simulink library "thc"  (R2021b)
settings: Solver=VariableStepAuto  StartTime=0.0  StopTime=10.0  RelTol=1e-3
undefined symbols (not defined in the file or in its folder): ATHC_APTCQA_X_C, ATHC_APTCQB_X_C, ATHC_dAy_X_C, ATHC_Qeq_X_kmh, ATHC_VbaseC_X_C, ATHC_VbaseC_Y_W, ATHC_VbaseD_X_C, ATHC_VbaseH_X_C, FALSE, KTHC_ACMaxMinT_sec, KTHC_aDeice_K, KTHC_AGSDefLv_K, KTHC_AGSLv1_K, KTHC_AGSLv2_K, KTHC_AGSLv3_K, KTHC_AGSLv4_K, KTHC_AGSLv5_K, KTHC_AirIntUpdateT_sec, KTHC_APTCOneZoneMax_W, KTHC_APTCQMaxC_W, KTHC_APTCQminC_W, KTHC_APTCQminD_W, KTHC_APTCQminRe1_W, KTHC_APTCQminRe_W, KTHC_APTCQoffT_cnt, KTHC_APTCQonT_cnt, KTHC_APTCRiLeMaxDff_W, KTHC_APTCRiLeMinDff_W, KTHC_BatInTempDef_C, KTHC_bDeice_K, KTHC_CompMaxDeice_rpm, KTHC_CompMinDeice_rpm, KTHC_CompSotxvOp_K, KTHC_CompSotxvOpLow_rpm, KTHC_CompSpdmax_rpm, KTHC_CompSpdmaxBC1_rpm, KTHC_CompSpdmaxBC_rpm, KTHC_CompSpdmid1_rpm, KTHC_CompSpdmid2_rpm, KTHC_CompSpdmid3_rpm, KTHC_CompSpdmid_rpm, KTHC_CompSpdmin_rpm, KTHC_DAPTCQ1_W, KTHC_DAPTCQ2_W, KTHC_DAPTCQ3_W, KTHC_DcChSetTemp_C, KTHC_DehumidityEN_flg, KTHC_DeiceCycTime_K, KTHC_DTambSat1_C, KTHC_DTambSat2_C, KTHC_DTambsat3_C, KTHC_DTambsat4_C, KTHC_DTambSat5_C, KTHC_DTambSat_C, KTHC_DTcabin10_C, KTHC_DTCabin11_C, KTHC_DTcabin12_C, KTHC_DTcabin1_C, KTHC_DTcabin2_C, KTHC_DTcabin3_C ... (+347)
libraries: simulink x80
(part 4 of 8)

== system thc/THC/ThermalControl/AC/ModMath2 ==
  Dividend : Inport
  Divisor : Inport  Port=2
  Abs : Abs
  Constant : Constant  Value=eps
  Data Type Conversion : DataTypeConversion
  Data Type Conversion1 : DataTypeConversion
  Data Type Conversion2 : DataTypeConversion  OutDataTypeStr=single
  Divide : Product  Inputs=*/
  Equal : RelationalOperator  Operator=<=  OutDataTypeStr=boolean  RndMeth=Simplest
  Floor : Rounding
  Minus : Sum  Inputs=+-
  Product : Product
  Switch : Switch  Criteria=u2 > Threshold
  Remainder : Outport
  wires:
  Divisor/1 -> [Divisor]
  Equal/1 -> Switch/2
  Constant/1 -> Equal/2
  [Dividend] -> Divide/1
  Switch/1 -> Remainder/1
  [Dividend] -> Switch/1
  Minus/1 -> Switch/3
  Data Type Conversion2/1 -> Floor/1
  Data Type Conversion/1 -> Minus/2
  [Dividend] -> Minus/1
  Dividend/1 -> [Dividend]
  Floor/1 -> Data Type Conversion1/1
  Data Type Conversion1/1 -> Product/1
  [Divisor] -> Divide/2
  Abs/1 -> Equal/1
  [Divisor] -> Product/2
  Divide/1 -> Data Type Conversion2/1
  Product/1 -> Data Type Conversion/1
  [Divisor] -> Abs/1

== system thc/THC/ThermalControl/THCM_Conctrl/AGSandFan ==
  AGSLV : Inport
  Fan_Err : Inport  Port=2
  FAN : Inport  Port=3
  Compare To Constant : simulink/Logic and Bit Operations/Compare To Constant  relop=>  const=1  OutDataTypeStr=boolean
  Constant : Constant  Value=KTHC_AGSLv1_K
  Constant1 : Constant  Value=KTHC_AGSLv2_K
  Constant2 : Constant  Value=KTHC_AGSLv3_K
  Constant3 : Constant  Value=KTHC_AGSLv4_K
  Constant4 : Constant  Value=KTHC_AGSLv5_K
  Constant5 : Constant  Value=0
  Constant6 : Constant  Value=KTHC_AGSDefLv_K
  Constant7 : Constant  Value=KTHC_ErrHandleEN_flg
  Logical Operator : Logic  Inputs=3  AllPortsSameDT=off  OutDataTypeStr=boolean
  Multiport Switch : MultiPortSwitch  Inputs=6  DiagnosticForDefault=None
  Switch : Switch  Criteria=u2 > Threshold
  AGSOut : Outport
  wires:
  Constant2/1 -> Multiport Switch/4
  Constant1/1 -> Multiport Switch/3
  Constant/1 -> Multiport Switch/2
  Constant3/1 -> Multiport Switch/5
  Constant4/1 -> Multiport Switch/6
  Constant5/1 -> Multiport Switch/7
  AGSLV/1 -> Multiport Switch/1
  FAN/1 -> Compare To Constant/1
  Fan_Err/1 -> Logical Operator/1
  Compare To Constant/1 -> Logical Operator/2
  Multiport Switch/1 -> Switch/3
  Logical Operator/1 -> Switch/2
  Switch/1 -> AGSOut/1
  Constant6/1 -> Switch/1
  Constant7/1 -> Logical Operator/3

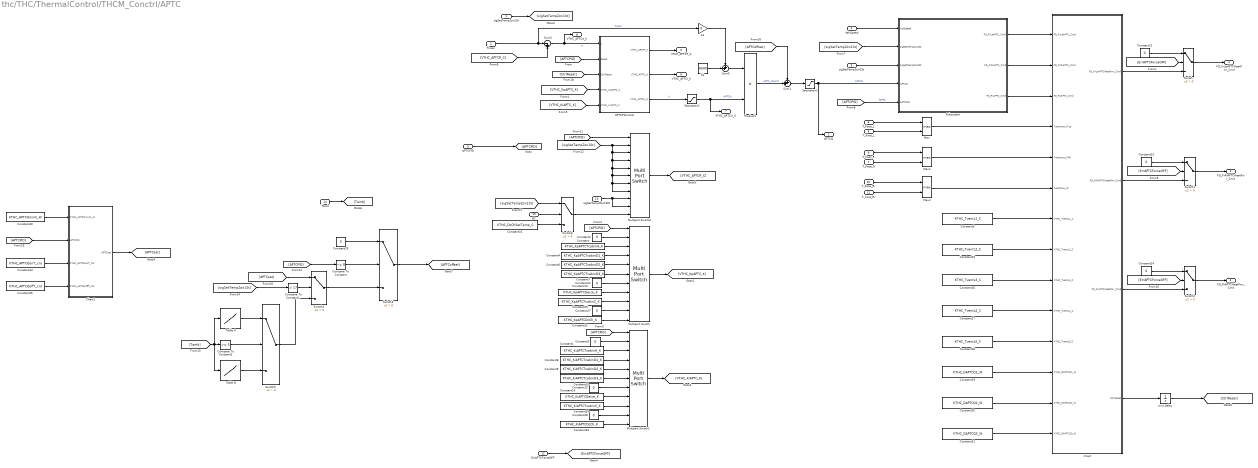
== system thc/THC/ThermalControl/THCM_Conctrl/APTC ==
  sigSetTempZon1St : Inport
  Tincar : Inport  Port=2
  APTCPID : Inport  Port=3
  VehSpeed : Inport  Port=4
  sigSetTempZon2St : Inport  Port=5
  T_Face_L : Inport  Port=6
  T_Face_R : Inport  Port=7
  T_Foot_L : Inport  Port=8
  T_Foot_R : Inport  Port=9
  T_Face_Rr : Inport  Port=10
  T_Foot_Rr : Inport  Port=11
  ErrAPTCForceOFF : Inport  Port=12
  sigSetTempZon1StC : Inport  Port=13
  Tamb : Inport  Port=14
  AC : Inport  Port=15
  APTCPIControl : Subsystem
  Chart : Stateflow chart  TreatAsAtomicUnit=on
  Chart1 : Stateflow chart  TreatAsAtomicUnit=on
  Compare To Constant : simulink/Logic and Bit Operations/Compare To Constant  relop=~=  const=8  OutDataTypeStr=boolean
  Compare To Constant1 : simulink/Logic and Bit Operations/Compare To Constant  relop=>  const=17  OutDataTypeStr=boolean
  Compare To Constant2 : simulink/Logic and Bit Operations/Compare To Constant  relop=>=  const=5  OutDataTypeStr=boolean
  Constant : Constant  Value=KTHC_KpAPTCTcabinH_K
  Constant1 : Constant  Value=KTHC_KiAPTCTcabinH_K
  Constant10 : Constant  Value=KTHC_KiAPTCTcabinD3_K
  Constant{2..3,11..12,22..24,27..29} (10 alike) : Constant  Value=0
  Constant13 : Constant  Value=KTHC_KpAPTCDeice_K
  Constant14 : Constant  Value=KTHC_KiAPTCDeice_K
  Constant15 : Constant  Value=KTHC_TventL2_C
  Constant16 : Constant  Value=KTHC_TventL3_C
  Constant17 : Constant  Value=KTHC_TventL4_C
  Constant18 : Constant  Value=KTHC_TventL5_C
  Constant19 : Constant  Value=KTHC_DAPTCQ1_W
  Constant20 : Constant  Value=KTHC_DAPTCQ2_W
  Constant21 : Constant  Value=KTHC_DAPTCQ3_W
  Constant25 : Constant  Value=KTHC_KpAPTCTcabinC_K
  Constant26 : Constant  Value=KTHC_KiAPTCTcabinC_K
  Constant30 : Constant  Value=KTHC_APTCQminC_W
  Constant31 : Constant  Value=KTHC_DcChSetTemp_C
  Constant32 : Constant  Value=KTHC_KpAPTCDcCh_K
  Constant33 : Constant  Value=KTHC_KiAPTCDcCh_K
  Constant34 : Constant  Value=KTHC_APTCQonT_cnt
  Constant35 : Constant  Value=KTHC_APTCQoffT_cnt
  Constant4 : Constant  Value=KTHC_KpAPTCTcabinD1_K
  Constant5 : Constant  Value=KTHC_TventL1_C
  Constant6 : Constant  Value=KTHC_KpAPTCTcabinD2_K
  Constant7 : Constant  Value=KTHC_KpAPTCTcabinD3_K
  Constant8 : Constant  Value=KTHC_KiAPTCTcabinD1_K
  Constant9 : Constant  Value=KTHC_KiAPTCTcabinD2_K
  Max : MinMax  Function=max  Inputs=2
  Max1 : MinMax  Function=max  Inputs=2
  Max2 : MinMax  Function=max  Inputs=2
  Multiport Switch : MultiPortSwitch  DataPortOrder=Zero-based contiguous  Inputs=10  zeroidx=on
  Multiport Switch1 : MultiPortSwitch  DataPortOrder=Zero-based contiguous  Inputs=10  zeroidx=on
  Multiport Switch2 : MultiPortSwitch  DataPortOrder=Zero-based contiguous  Inputs=10  zeroidx=on
  Product1 : Product
  Saturation1 : Saturate  UpperLimit=1  LowerLimit=0
  Saturation2 : Saturate  UpperLimit=6500  LowerLimit=0
  Subsystem : Subsystem
  Sum1 : Sum  Inputs=++|
  Sum3 : Sum  Inputs=|-+
  Sum5 : Sum  Inputs=++|
  Switch{,1..6} (7 alike) : Switch  Criteria=u2 > Threshold
  Table A : Lookup_n-D  NumberOfTableDimensions=1  BreakpointsForDimension1=ATHC_APTCQA_X_C  Table=MTHC_APTCQA_Y_W  InternalRulePriority=Speed  RndMeth=Simplest  InputSameDT=on
  Table B : Lookup_n-D  NumberOfTableDimensions=1  BreakpointsForDimension1=ATHC_APTCQB_X_C  Table=MTHC_APTCQB_Y_W  InternalRulePriority=Speed  RndMeth=Simplest  InputSameDT=on
  Unit Delay : UnitDelay  SampleTime=-1  HasFrameUpgradeWarning=on
  a1 : Gain  Gain=0
  b1 : Constant  Value=6500
  APTCQ : Outport
  FD_FrLeAPTCHeatPwr_Cmd : Outport  Port=2
  FD_FrRiAPTCHeatPwr_Cmd : Outport  Port=3
  FD_RrAPTCHeatPwr_Cmd : Outport  Port=4
  VTHC_APTCP_K : Outport  Port=5
  VTHC_APTCI_K : Outport  Port=6
  VTHC_APTCU_K : Outport  Port=7
  VTHC_APTCe_K : Outport  Port=8
  wires:
  [VTHC_APTCR_C] -> Sum3/2
  a1/1 -> Sum5/1
  Product1/1 -> Sum1/2  "APTC_nolimit"
  Saturation1/1 -> VTHC_APTCU_K/1, Product1/2  "APTC%"
  Tincar/1 -> a1/1, Sum3/1  "Tincar"
  Sum5/1 -> Product1/1
  b1/1 -> Sum5/2
  Sum3/1 -> VTHC_APTCe_K/1, APTCPIControl/1(x)  "e"
  APTCPIControl/3(VTHC_APTCU_K) -> Saturation1/1  "U"
  [APTCPID] -> APTCPIControl/2(Reset)
  Saturation2/1 -> APTCQ/1, Subsystem/4(APTCQ)  "APTCQ"
  Constant/1 -> Multiport Switch/3
  Constant1/1 -> Multiport Switch1/3
  APTCPIControl/1(VTHC_APTCP_K) -> VTHC_APTCP_K/1
  APTCPIControl/2(VTHC_APTCI_K) -> VTHC_APTCI_K/1
  [APTCPID] -> Multiport Switch/1
  Constant2/1 -> Multiport Switch/2
  Multiport Switch/1 -> [VTHC_KpAPTC_K]
  Multiport Switch1/1 -> [VTHC_KiAPTC_K]
  Constant3/1 -> Multiport Switch1/2
  [APTCPID] -> Multiport Switch1/1
  Constant4/1 -> Multiport Switch/4
  Constant6/1 -> Multiport Switch/5
  Constant7/1 -> Multiport Switch/6
  Constant8/1 -> Multiport Switch1/4
  Constant9/1 -> Multiport Switch1/5
  Constant10/1 -> Multiport Switch1/6
  [VTHC_KpAPTC_K] -> APTCPIControl/4(VTHC_KpAPTC_K)
  [VTHC_KiAPTC_K] -> APTCPIControl/5(VTHC_KiAPTC_K)
  Constant11/1 -> Multiport Switch/7
  Constant12/1 -> Multiport Switch1/7
  VehSpeed/1 -> Subsystem/1(VehSpeed)
  sigSetTempZon2St/1 -> Subsystem/3(sigSetTempZon2St)
  [sigSetTempZon1St] -> Subsystem/2(sigSetTempZon1St)
  sigSetTempZon1St/1 -> [sigSetTempZon1St]
  [APTCPID] -> Subsystem/5(APTCPID)  "fAPTC"
  Constant13/1 -> Multiport Switch/8
  Constant14/1 -> Multiport Switch1/8
  T_Face_Rr/1 -> Max2/1
  T_Foot_L/1 -> Max/2
  T_Face_L/1 -> Max/1
  T_Foot_R/1 -> Max1/1
  T_Face_R/1 -> Max1/2
  T_Foot_Rr/1 -> Max2/2
  Max/1 -> Chart/4(Tventmax_FrLe)
  Subsystem/1(FD_FrLeAPTC_Cmd) -> Chart/1(FD_FrLeAPTC_Cmd)
  Subsystem/2(FD_FrRiAPTC_Cmd) -> Chart/2(FD_FrRiAPTC_Cmd)
  Subsystem/3(FD_RrAPTC_Cmd) -> Chart/3(FD_RrAPTC_Cmd)
  Max1/1 -> Chart/5(Tventmax_FrRi)
  Max2/1 -> Chart/6(Tventmax_Rr)
  Constant5/1 -> Chart/7(KTHC_TventL1_C)
  Constant15/1 -> Chart/8(KTHC_TventL2_C)
  Constant16/1 -> Chart/9(KTHC_TventL3_C)
  Constant17/1 -> Chart/10(KTHC_TventL4_C)
  Constant18/1 -> Chart/11(KTHC_TventL5_C)
  Constant19/1 -> Chart/12(KTHC_DAPTCQ1_W)
  Constant20/1 -> Chart/13(KTHC_DAPTCQ2_W)
  Constant21/1 -> Chart/14(KTHC_DAPTCQ3_W)
  Chart/1(FD_FrLeAPTCHeatPwr_Cmd) -> Switch/3
  ErrAPTCForceOFF/1 -> [ErrAPTCForceOFF]
  Switch/1 -> FD_FrLeAPTCHeatPwr_Cmd/1
  [ErrAPTCForceOFF] -> Switch/2
  Constant22/1 -> Switch/1
  Constant23/1 -> Switch1/1
  [ErrAPTCForceOFF] -> Switch1/2
  Chart/2(FD_FrRiAPTCHeatPwr_Cmd) -> Switch1/3
  Switch1/1 -> FD_FrRiAPTCHeatPwr_Cmd/1
  Chart/3(FD_RrAPTCHeatPwr_Cmd) -> Switch2/3
  [ErrAPTCForceOFF] -> Switch2/2
  Constant24/1 -> Switch2/1
  Switch2/1 -> FD_RrAPTCHeatPwr_Cmd/1
  Multiport Switch2/1 -> [VTHC_APTCR_C]
  [APTCPID] -> Multiport Switch2/1
  [sigSetTempZon1St] -> Multiport Switch2/8, Multiport Switch2/7, Multiport Switch2/6, Multiport Switch2/5, Multiport Switch2/4, Multiport Switch2/3, Multiport Switch2/2
  Constant25/1 -> Multiport Switch/9
  Constant26/1 -> Multiport Switch1/9
  APTCPID/1 -> [APTCPID]
  sigSetTempZon1StC/1 -> Multiport Switch2/10, Multiport Switch2/9
  Constant27/1 -> Multiport Switch/10
  Constant28/1 -> Multiport Switch1/10
  [APTCPID] -> Compare To Constant/1
  [sigSetTempZon1St] -> Compare To Constant1/1
  Compare To Constant1/1 -> Switch4/2
  Compare To Constant/1 -> Switch3/2
  Constant29/1 -> Switch3/1
  Switch4/1 -> Switch3/3
  Tamb/1 -> [Tamb]
  [Tamb] -> Table B/1, Table A/1, Compare To Constant2/1
  Compare To Constant2/1 -> Switch5/2
  Table A/1 -> Switch5/1
  Table B/1 -> Switch5/3
  Switch5/1 -> Switch4/3
  Switch3/1 -> [APTCoffset]
  Sum1/1 -> Saturation2/1
  [APTCoffset] -> Sum1/1
  AC/1 -> Switch6/2
  [sigSetTempZon1St] -> Switch6/1
  Constant31/1 -> Switch6/3
  Switch6/1 -> Multiport Switch2/11
  Constant32/1 -> Multiport Switch/11
  Constant33/1 -> Multiport Switch1/11
  Chart/4(CtrlReset) -> Unit Delay/1
  Unit Delay/1 -> [CtrlReset]
  [CtrlReset] -> APTCPIControl/3(CtrlReset)
  Constant30/1 -> Chart1/1(KTHC_APTCQminC_W)
  [APTCPID] -> Chart1/2(APTCPID)
  Constant34/1 -> Chart1/3(KTHC_APTCQonT_cnt)
  Constant35/1 -> Chart1/4(KTHC_APTCQoffT_cnt)
  Chart1/1(APTCset) -> [APTCset]
  [APTCset] -> Switch4/1

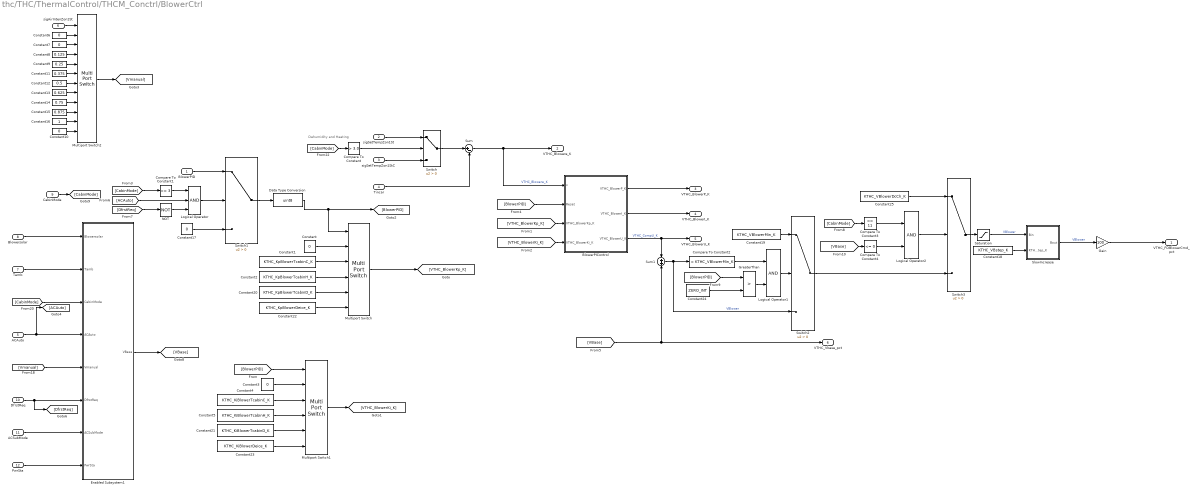
== system thc/THC/ThermalControl/THCM_Conctrl/BlowerCtrl ==
  note: Dehumidity and Heating
  BlowerPID : Inport
  sigSetTempZon1St : Inport  Port=2
  sigSetTempZon1StC : Inport  Port=3
  Tincar : Inport  Port=4
  ACAuto : Inport  Port=5
  sigAirIntenZon1St : Inport  Port=6
  Tamb : Inport  Port=7
  Blowersolar : Inport  Port=8
  CabinMode : Inport  Port=9
  DfrstReq : Inport  Port=10
  ACSubMode : Inport  Port=11
  PwrSta : Inport  Port=12
  BlowerPIControl : Subsystem
  Compare To Constant : simulink/Logic and Bit Operations/Compare To Constant  relop=>  const=3.0  OutDataTypeStr=boolean
  Compare To Constant1 : simulink/Logic and Bit Operations/Compare To Constant  relop=>=  const=3  OutDataTypeStr=boolean
  Compare To Constant2 : simulink/Logic and Bit Operations/Compare To Constant  relop=<  const=KTHC_VBlowerMin_K  OutDataTypeStr=boolean
  Compare To Constant3 : simulink/Logic and Bit Operations/Compare To Constant  relop===  const=11  OutDataTypeStr=boolean
  Compare To Constant4 : simulink/Logic and Bit Operations/Compare To Constant  relop=<=  const=0  OutDataTypeStr=boolean
  Constant{,3,6..7,10,17} (6 alike) : Constant  Value=0
  Constant1 : Constant  Value=KTHC_KpBlowerTcabinC_K
  Constant11 : Constant  Value=0.375
  Constant12 : Constant  Value=0.5
  Constant13 : Constant  Value=0.625
  Constant14 : Constant  Value=0.75
  Constant15 : Constant  Value=0.875
  Constant16 : Constant
  Constant18 : Constant  Value=KTHC_VBstep_K
  Constant19 : Constant  Value=KTHC_VBlowerMin_K
  Constant2 : Constant  Value=KTHC_KpBlowerTcabinH_K
  Constant20 : Constant  Value=KTHC_KpBlowerTcabinD_K
  Constant21 : Constant  Value=KTHC_KiBlowerTcabinD_K
  Constant22 : Constant  Value=KTHC_KpBlowerDeice_K
  Constant23 : Constant  Value=KTHC_KiBlowerDeice_K
  Constant24 : Constant  Value=ZERO_INT
  Constant25 : Constant  Value=KTHC_VBlowerDcCh_K
  Constant4 : Constant  Value=KTHC_KiBlowerTcabinC_K
  Constant5 : Constant  Value=KTHC_KiBlowerTcabinH_K
  Constant8 : Constant  Value=0.125
  Constant9 : Constant  Value=0.25
  Data Type Conversion : DataTypeConversion  OutDataTypeStr=uint8
  Enabled Subsystem1 : Subsystem  TreatAsAtomicUnit=on
  Gain : Gain  Gain=100
  GreaterThan : RelationalOperator  Operator=>  OutDataTypeStr=boolean  RndMeth=Simplest
  Logical Operator : Logic  Inputs=3  AllPortsSameDT=off  OutDataTypeStr=boolean
  Logical Operator1 : Logic  AllPortsSameDT=off  OutDataTypeStr=boolean
  Logical Operator2 : Logic  AllPortsSameDT=off  OutDataTypeStr=boolean
  Multiport Switch : MultiPortSwitch  DataPortOrder=Zero-based contiguous  Inputs=5  zeroidx=on
  Multiport Switch1 : MultiPortSwitch  DataPortOrder=Zero-based contiguous  Inputs=5  zeroidx=on
  Multiport Switch2 : MultiPortSwitch  DataPortOrder=Zero-based contiguous  Inputs=11  zeroidx=on
  NOT : Logic  Operator=NOT  IconShape=distinctive  AllPortsSameDT=off  OutDataTypeStr=boolean
  Saturation : Saturate  UpperLimit=1  LowerLimit=0
  SlowIncrease : Stateflow chart  TreatAsAtomicUnit=on
  Sum : Sum  Inputs=|+-
  Sum1 : Sum  Inputs=+|+
  Switch{,1..3} (4 alike) : Switch  Criteria=u2 > Threshold
  VTHC_FDBlowerCmd_pct : Outport
  VTHC_Blowere_K : Outport  Port=2
  VTHC_BlowerP_K : Outport  Port=3
  VTHC_BlowerI_K : Outport  Port=4
  VTHC_BlowerU_K : Outport  Port=5
  VTHC_Vbase_pct : Outport  Port=6
  wires:
  CabinMode/1 -> [CabinMode]
  Tamb/1 -> Enabled Subsystem1/2(Tamb)
  Multiport Switch2/1 -> [Vmanual]
  Blowersolar/1 -> Enabled Subsystem1/1(Blowersolar)
  Constant12/1 -> Multiport Switch2/7
  Constant7/1 -> Multiport Switch2/3
  Constant9/1 -> Multiport Switch2/5
  Constant14/1 -> Multiport Switch2/9
  Constant15/1 -> Multiport Switch2/10
  sigAirIntenZon1St/1 -> Multiport Switch2/1
  [Vmanual] -> Enabled Subsystem1/5(Vmanual)
  Multiport Switch/1 -> [VTHC_BlowerKp_K]
  Switch/1 -> Sum/1
  ACAuto/1 -> [ACAuto], Enabled Subsystem1/4(ACAuto)
  BlowerPIControl/2(VTHC_BlowerI_K) -> VTHC_BlowerI_K/1
  [VTHC_BlowerKp_K] -> BlowerPIControl/3(VTHC_BlowerKp_K)
  Constant8/1 -> Multiport Switch2/4
  Sum/1 -> VTHC_Blowere_K/1, BlowerPIControl/1(x)  "VTHC_Blowere_K"
  Sum1/1 -> Compare To Constant2/1, Switch2/3  "VBlower"
  [VBase] -> VTHC_Vbase_pct/1, Sum1/2
  sigSetTempZon1St/1 -> Switch/1
  Constant13/1 -> Multiport Switch2/8
  Constant4/1 -> Multiport Switch1/3
  Constant16/1 -> Multiport Switch2/11
  Tincar/1 -> Sum/2
  BlowerPIControl/1(VTHC_BlowerP_K) -> VTHC_BlowerP_K/1
  Constant11/1 -> Multiport Switch2/6
  Data Type Conversion/1 -> Multiport Switch/1, [BlowerPID]
  Constant3/1 -> Multiport Switch1/2
  Constant/1 -> Multiport Switch/2
  [BlowerPID] -> Multiport Switch1/1
  sigSetTempZon1StC/1 -> Switch/3
  Multiport Switch1/1 -> [VTHC_BlowerKi_K]
  [BlowerPID] -> BlowerPIControl/2(Reset)
  Constant10/1 -> Multiport Switch2/12
  Constant2/1 -> Multiport Switch/4
  BlowerPIControl/3(VTHC_BlowerU_K) -> VTHC_BlowerU_K/1, Sum1/1  "VTHC_CompU_K"
  [VTHC_BlowerKi_K] -> BlowerPIControl/4(VTHC_BlowerKi_K)
  Constant6/1 -> Multiport Switch2/2
  Enabled Subsystem1/1(VBase) -> [VBase]
  Constant1/1 -> Multiport Switch/3
  Constant5/1 -> Multiport Switch1/4
  Gain/1 -> VTHC_FDBlowerCmd_pct/1
  DfrstReq/1 -> [DfrstReq], Enabled Subsystem1/6(DfrstReq)
  [CabinMode] -> Enabled Subsystem1/3(CabinMode)
  [CabinMode] -> Compare To Constant/1
  Compare To Constant/1 -> Switch/2
  Constant20/1 -> Multiport Switch/5
  Constant21/1 -> Multiport Switch1/5
  SlowIncrease/1(Bout) -> Gain/1  "VBlower"
  ACSubMode/1 -> Enabled Subsystem1/7(ACSubMode)
  BlowerPID/1 -> Switch1/1
  Compare To Constant1/1 -> Logical Operator/1
  [CabinMode] -> Compare To Constant1/1
  Constant17/1 -> Switch1/3
  Logical Operator/1 -> Switch1/2
  [ACAuto] -> Logical Operator/2
  [DfrstReq] -> NOT/1
  NOT/1 -> Logical Operator/3
  PwrSta/1 -> Enabled Subsystem1/8(PwrSta)
  Saturation/1 -> SlowIncrease/1(Bin)  "VBlower"
  Constant18/1 -> SlowIncrease/2(KTHC_VBstep_K)
  [BlowerPID] -> GreaterThan/1
  Compare To Constant2/1 -> Logical Operator1/1
  Logical Operator1/1 -> Switch2/2
  Constant19/1 -> Switch2/1
  Constant22/1 -> Multiport Switch/6
  Constant23/1 -> Multiport Switch1/6
  Switch1/1 -> Data Type Conversion/1
  Constant24/1 -> GreaterThan/2
  GreaterThan/1 -> Logical Operator1/2
  Switch2/1 -> Switch3/3
  Switch3/1 -> Saturation/1
  [CabinMode] -> Compare To Constant3/1
  Constant25/1 -> Switch3/1
  Logical Operator2/1 -> Switch3/2
  Compare To Constant3/1 -> Logical Operator2/1
  Compare To Constant4/1 -> Logical Operator2/2
  [VBase] -> Compare To Constant4/1

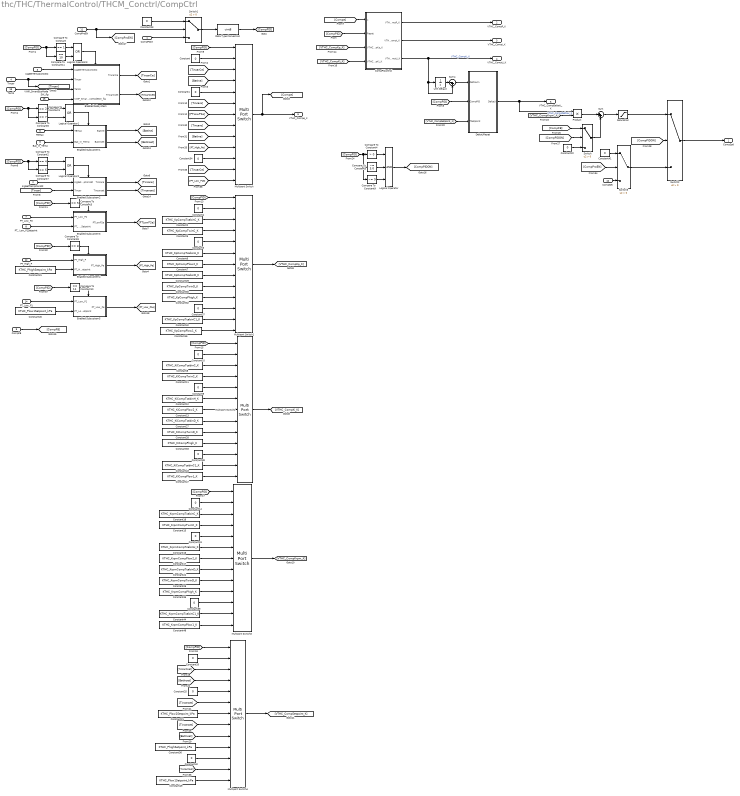
== system thc/THC/ThermalControl/THCM_Conctrl/CompCtrl ==
  CompPIDin : Inport
  sigSetTempZon1St : Inport  Port=2
  sigSetTempZon1StC : Inport  Port=3
  Tincar : Inport  Port=4
  TBMax : Inport  Port=5
  Bat_In_Temp : Inport  Port=6
  PT_Low_P2 : Inport  Port=7
  PT_ Low_P2Setpoint : Inport  Port=8
  CompFB : Inport  Port=9
  CompSet : Inport  Port=10
  CompProEN : Inport  Port=11
  PT_High_P : Inport  Port=12
  Tamb : Inport  Port=13
  PT_Low_P1 : Inport  Port=14
  VINP_SmartEcoModeSW_flg : Inport  Port=15
  CompPIControl : Subsystem
  Compare To Constant : simulink/Logic and Bit Operations/Compare To Constant  relop===  const=1  OutDataTypeStr=boolean
  Compare To Constant1 : simulink/Logic and Bit Operations/Compare To Constant  relop===  const=2  OutDataTypeStr=boolean
  Compare To Constant10 : simulink/Logic and Bit Operations/Compare To Constant  relop===  const=11  OutDataTypeStr=boolean
  Compare To Constant11 : simulink/Logic and Bit Operations/Compare To Constant  relop===  const=10  OutDataTypeStr=boolean
  Compare To Constant2 : simulink/Logic and Bit Operations/Compare To Constant  relop===  const=4  OutDataTypeStr=boolean
  Compare To Constant3 : simulink/Logic and Bit Operations/Compare To Constant  relop===  const=5  OutDataTypeStr=boolean
  Compare To Constant4 : simulink/Logic and Bit Operations/Compare To Constant  relop=>  const=0  OutDataTypeStr=boolean
  Compare To Constant5 : simulink/Logic and Bit Operations/Compare To Constant  relop=~=  const=3.0  OutDataTypeStr=boolean
  Compare To Constant6 : simulink/Logic and Bit Operations/Compare To Constant  relop===  const=7  OutDataTypeStr=boolean
  Compare To Constant7 : simulink/Logic and Bit Operations/Compare To Constant  relop===  const=6  OutDataTypeStr=boolean
  Compare To Constant8 : simulink/Logic and Bit Operations/Compare To Constant  relop===  const=8  OutDataTypeStr=boolean
  Compare To Constant9 : simulink/Logic and Bit Operations/Compare To Constant  relop=~=  const=9  OutDataTypeStr=boolean
  Constant{,1,3..4,9..10,14,19..20,22..23,25,34,37..41} (18 alike) : Constant  Value=0
  Constant11 : Constant  Value=KTHC_KiCompTwinC_K
  Constant12 : Constant  Value=KTHC_KiCompTcabinH_K
  Constant13 : Constant  Value=KTHC_KiCompPlow2_K
  Constant15 : Constant  Value=KTHC_KrpmCompTwinC_K
  Constant16 : Constant  Value=KTHC_KrpmCompTcabinH_K
  Constant17 : Constant  Value=KTHC_KrpmCompPlow2_K
  Constant18 : Constant  Value=KTHC_KrpmCompTcabinC_K
  Constant2 : Constant  Value=KTHC_KpCompTcabinC_K
  Constant21 : Constant  Value=KTHC_Plow2Setpoint_kPa
  Constant24 : Constant  Value=KTHC_KrpmCompTcabinD_K
  Constant26 : Constant  Value=KTHC_KrpmCompTwinD_K
  Constant27 : Constant  Value=KTHC_KiCompTcabinD_K
  Constant28 : Constant  Value=KTHC_KiCompTwinD_K
  Constant29 : Constant  Value=KTHC_KpCompTcabinD_K
  Constant30 : Constant  Value=KTHC_KpCompTwinD_K
  Constant31 : Constant  Value=KTHC_PhighSetpoint_kPa
  Constant32 : Constant  Value=KTHC_KpCompPhigh_K
  Constant33 : Constant  Value=KTHC_KiCompPhigh_K
  Constant35 : Constant  Value=KTHC_KrpmCompPhigh_K
  Constant36 : Constant  Value=KTHC_PhighSetpoint_kPa
  Constant42 : Constant  Value=KTHC_KpCompTcabinC1_K
  Constant43 : Constant  Value=KTHC_KiCompTcabinC1_K
  Constant44 : Constant  Value=KTHC_KrpmCompTcabinC1_K
  Constant45 : Constant  Value=KTHC_Plow1Setpoint_kPa
  Constant46 : Constant  Value=KTHC_KpCompPlow1_K
  Constant47 : Constant  Value=KTHC_KiCompPlow1_K
  Constant48 : Constant  Value=KTHC_KrpmCompPlow1_K
  Constant49 : Constant  Value=KTHC_Plow1Setpoint_kPa
  Constant5 : Constant  Value=KTHC_KpCompTwinC_K
  Constant6 : Constant  Value=KTHC_KpCompTcabinH_K
  Constant7 : Constant  Value=KTHC_KpCompPlow2_K
  Constant8 : Constant  Value=KTHC_KiCompTcabinC_K
  Data Type Conversion : DataTypeConversion  OutDataTypeStr=uint8
  DeltaUReset : Subsystem
  Enabled Subsystem : Subsystem  TreatAsAtomicUnit=on
  Enabled Subsystem1 : Subsystem  TreatAsAtomicUnit=on
  Enabled Subsystem2 : Subsystem  TreatAsAtomicUnit=on
  Enabled Subsystem3 : Subsystem  TreatAsAtomicUnit=on
  Enabled Subsystem4 : Subsystem  TreatAsAtomicUnit=on
  Enabled Subsystem5 : Subsystem  TreatAsAtomicUnit=on
  Logical Operator : Logic  Inputs=3  AllPortsSameDT=off  OutDataTypeStr=boolean
  Logical Operator1 : Logic  Operator=OR  AllPortsSameDT=off  OutDataTypeStr=boolean
  Logical Operator2 : Logic  Operator=OR  AllPortsSameDT=off  OutDataTypeStr=boolean
  Logical Operator3 : Logic  Operator=OR  AllPortsSameDT=off  OutDataTypeStr=boolean
  Multiport Switch{,1..4} (5 alike) : MultiPortSwitch  DataPortOrder=Zero-based contiguous  Inputs=12  DiagnosticForDefault=None  zeroidx=on
  Product : Product
  Saturation : Saturate  UpperLimit=KTHC_CompSpdmax_rpm  LowerLimit=KTHC_CompSpdmin_rpm  OutDataTypeStr=double
  Sum : Sum  Inputs=|++
  Sum4 : Sum  Inputs=|-+
  Switch{,1..3} (4 alike) : Switch  Criteria=u2 > Threshold
  Unit Delay2 : UnitDelay  SampleTime=-1  HasFrameUpgradeWarning=on
  CompSpd : Outport
  VTHC_CompP_K : Outport  Port=2
  VTHC_CompI_K : Outport  Port=3
  VTHC_CompU_K : Outport  Port=4
  VTHC_CompDeltaU_K : Outport  Port=5
  VTHC_Compe_K : Outport  Port=6
  wires:
  [CompPID] -> Compare To Constant9/1, Compare To Constant5/1, Compare To Constant4/1
  Constant22/1 -> Switch/3
  Switch/1 -> Sum/2
  Multiport Switch4/1 -> [VTHC_CompSetpoint_K]
  [CompPID] -> Multiport Switch4/1
  Constant25/1 -> Multiport Switch4/5
  Constant20/1 -> Multiport Switch4/2
  Constant12/1 -> Multiport Switch2/6
  [CompPID] -> Multiport Switch2/1
  Constant9/1 -> Multiport Switch2/5
  Multiport Switch2/1 -> [VTHC_CompKi_K]
  Constant13/1 -> Multiport Switch2/7
  Constant10/1 -> Multiport Switch2/2
  Constant5/1 -> Multiport Switch1/4
  Constant7/1 -> Multiport Switch1/7
  PT_ Low_P2Setpoint/1 -> Enabled Subsystem3/2(PT_ Low_P2Setpoint)
  [BatInset] -> Multiport Switch4/4
  sigSetTempZon1St/1 -> Enabled Subsystem2/1(sigSetTempZon1St)
  Constant3/1 -> Multiport Switch1/5
  Constant1/1 -> Multiport Switch/5
  Compare To Constant1/1 -> Logical Operator1/1
  [Compe] -> CompPIControl/1(x)
  CompFB/1 -> [CompFB]
  [BatIne] -> Multiport Switch/4
  Product/1 -> Sum/1
  Enabled Subsystem1/2(BatInset) -> [BatInset]
  Enabled Subsystem2/2(Tincarset) -> [Tincarset]
  [VTHC_CompKp_K] -> CompPIControl/3(VTHC_CompKp_K)
  Constant2/1 -> Multiport Switch1/3
  Constant8/1 -> Multiport Switch2/3
  Bat_In_Temp/1 -> Enabled Subsystem1/2(Bat_In_Temp)
  Unit Delay2/1 -> Sum4/1
  [CompPID] -> DeltaUReset/2(CompPID)
  [CompPID] -> Compare To Constant3/1
  Constant/1 -> Multiport Switch/2
  Tincar/1 -> [Tincar], Enabled Subsystem/2(Tincar)
  [TincarCe] -> Multiport Switch/3
  [CompPID] -> CompPIControl/2(Reset)
  Compare To Constant3/1 -> Enabled Subsystem3/Enable
  [Tincar] -> Enabled Subsystem2/2(Tincar)
  Switch2/1 -> CompSpd/1
  [Tincarset] -> Multiport Switch4/6
  Multiport Switch/1 -> [Compe], VTHC_Compe_K/1
  Sum/1 -> Saturation/1
  Saturation/1 -> Switch2/1
  [VTHC_CompKrpm_K] -> Product/2
  Compare To Constant/1 -> Logical Operator3/1
  [CompPID] -> Compare To Constant6/1, Compare To Constant1/1
  [CompPIDON] -> Switch2/2
  CompPIControl/2(VTHC_CompI_K) -> VTHC_CompI_K/1
  [VTHC_CompSetpoint_K] -> DeltaUReset/3(TSetpoint)
  Compare To Constant4/1 -> Logical Operator/1
  Logical Operator/1 -> [CompPIDON]
  Constant4/1 -> Multiport Switch1/2
  sigSetTempZon1StC/1 -> Enabled Subsystem/1(sigSetTempZon1StC)
  Compare To Constant5/1 -> Logical Operator/2
  [CompPIDON] -> Switch/2
  Constant14/1 -> Multiport Switch3/2
  Constant17/1 -> Multiport Switch3/7
  Sum4/1 -> DeltaUReset/1(DeltaUin)
  Constant16/1 -> Multiport Switch3/6
  [VTHC_CompKi_K] -> CompPIControl/4(VTHC_CompKi_K)
  Multiport Switch3/1 -> [VTHC_CompKrpm_K]
  TBMax/1 -> Enabled Subsystem1/1(TBMax)
  Constant18/1 -> Multiport Switch3/3
  [CompPID] -> Compare To Constant11/1, Compare To Constant/1
  Constant19/1 -> Multiport Switch3/5
  CompSet/1 -> Switch3/3
  CompPIControl/3(VTHC_CompU_K) -> Sum4/2, Unit Delay2/1, VTHC_CompU_K/1  "VTHC_CompU_K"
  [CompPID] -> Multiport Switch3/1
  DeltaUReset/1(DeltaU) -> VTHC_CompDeltaU_K/1, Product/1  "VTHC_CompDeltaU_K"
  [CompPID] -> Multiport Switch1/1
  Multiport Switch1/1 -> [VTHC_CompKp_K]
  Constant21/1 -> Multiport Switch4/7
  Enabled Subsystem2/1(Tincare) -> [Tincare]
  Constant6/1 -> Multiport Switch1/6
  PT_Low_P2/1 -> Enabled Subsystem3/1(PT_Low_P2)
  Enabled Subsystem3/1(PTLowP2e) -> [PTLowP2e]
  Constant15/1 -> Multiport Switch3/4
  Enabled Subsystem/1(TincarCe) -> [TincarCe]
  [PTLowP2e] -> Multiport Switch/7
  [CompFB] -> Switch/1
  Enabled Subsystem/2(TincarCset) -> [TincarCset]
  Enabled Subsystem1/1(BatIne) -> [BatIne]
  CompPIControl/1(VTHC_CompP_K) -> VTHC_CompP_K/1
  Constant11/1 -> Multiport Switch2/4
  [Tincare] -> Multiport Switch/6
  CompPIDin/1 -> Switch1/3
  [TincarCset] -> Multiport Switch4/3
  [CompPID] -> Multiport Switch/1
  CompProEN/1 -> [CompProEN], Switch1/2
  Constant23/1 -> Switch1/1
  Switch1/1 -> Data Type Conversion/1
  Compare To Constant6/1 -> Logical Operator1/2
  Logical Operator1/1 -> Enabled Subsystem1/Enable
  Logical Operator2/1 -> Enabled Subsystem2/Enable
  Compare To Constant7/1 -> Logical Operator2/2
  [CompPID] -> Compare To Constant2/1, Compare To Constant7/1
  Compare To Constant2/1 -> Logical Operator2/1
  [Tincarset] -> Multiport Switch4/8
  [BatInset] -> Multiport Switch4/9
  Constant24/1 -> Multiport Switch3/8
  Constant26/1 -> Multiport Switch3/9
  Constant27/1 -> Multiport Switch2/8
  Constant28/1 -> Multiport Switch2/9
  Constant29/1 -> Multiport Switch1/8
  Constant30/1 -> Multiport Switch1/9
  [Tincare] -> Multiport Switch/8
  [BatIne] -> Multiport Switch/9
  Enabled Subsystem4/1(PT_High_Pe) -> [PT_High_Pe]
  PT_High_P/1 -> Enabled Subsystem4/1(PT_High_P)
  Compare To Constant8/1 -> Enabled Subsystem4/Enable
  [CompPID] -> Compare To Constant8/1
  Constant31/1 -> Enabled Subsystem4/2(PT_High_PSetpoint)
  [PT_High_Pe] -> Multiport Switch/10
  Constant32/1 -> Multiport Switch1/10
  Constant33/1 -> Multiport Switch2/10
  Constant36/1 -> Multiport Switch4/10
  Constant35/1 -> Multiport Switch3/10
  Constant34/1 -> Multiport Switch/11
  Constant37/1 -> Multiport Switch1/11
  Constant38/1 -> Multiport Switch2/11
  Constant39/1 -> Multiport Switch3/11
  Compare To Constant9/1 -> Logical Operator/3
  Constant40/1 -> Multiport Switch4/11
  Switch3/1 -> Switch2/3
  Constant41/1 -> Switch3/1
  [CompProEN] -> Switch3/2
  Tamb/1 -> Enabled Subsystem/3(Tamb)
  Data Type Conversion/1 -> [CompPID]
  [TincarCe] -> Multiport Switch/12
  Constant42/1 -> Multiport Switch1/12
  Constant43/1 -> Multiport Switch2/12
  Constant44/1 -> Multiport Switch3/12
  [TincarCset] -> Multiport Switch4/12
  Constant45/1 -> Enabled Subsystem5/2(PT_Low_P1Setpoint)
  [CompPID] -> Compare To Constant10/1
  Compare To Constant10/1 -> Enabled Subsystem5/Enable
  PT_Low_P1/1 -> Enabled Subsystem5/1(PT_Low_P1)
  Enabled Subsystem5/1(PT_Low_Pe) -> [PT_Low_P1e]
  [PT_Low_P1e] -> Multiport Switch/13
  Constant46/1 -> Multiport Switch1/13
  Constant47/1 -> Multiport Switch2/13
  Constant48/1 -> Multiport Switch3/13
  Constant49/1 -> Multiport Switch4/13
  Logical Operator3/1 -> Enabled Subsystem/Enable
  Compare To Constant11/1 -> Logical Operator3/2
  VINP_SmartEcoModeSW_flg/1 -> Enabled Subsystem/4(VINP_SmartEcoModeSW_flg)

== system thc/THC/ThermalControl/THCM_Conctrl/EWP1 ==
  EWPLV : Inport
  Constant : Constant  Value=KTHC_EWPLv1_K
  Constant1 : Constant  Value=KTHC_EWPLv2_K
  Constant2 : Constant  Value=KTHC_EWPLv3_K
  Constant3 : Constant  Value=KTHC_EWPLv4_K
  Constant4 : Constant  Value=KTHC_EWPLv5_K
  Constant5 : Constant  Value=0
  Constant6 : Constant  Value=KTHC_EWP3SpdDeice_K
  Constant7 : Constant  Value=125
  Constant8 : Constant  Value=KTHC_EWPDcCharge_K
  Multiport Switch : MultiPortSwitch  Inputs=9  DiagnosticForDefault=None
  EWPOut : Outport
  wires:
  Constant7/1 -> Multiport Switch/8
  EWPLV/1 -> Multiport Switch/1
  Constant5/1 -> Multiport Switch/10
  Constant4/1 -> Multiport Switch/6
  Constant3/1 -> Multiport Switch/5
  Constant/1 -> Multiport Switch/2
  Constant1/1 -> Multiport Switch/3
  Constant2/1 -> Multiport Switch/4
  Multiport Switch/1 -> EWPOut/1
  Constant6/1 -> Multiport Switch/7
  Constant8/1 -> Multiport Switch/9

== system thc/THC/ThermalControl/THCM_Conctrl/EWP2 ==
  EWPLV : Inport
  Constant : Constant  Value=KTHC_EWPLv1_K
  Constant1 : Constant  Value=KTHC_EWPLv2_K
  Constant2 : Constant  Value=KTHC_EWPLv3_K
  Constant3 : Constant  Value=KTHC_EWPLv4_K
  Constant4 : Constant  Value=KTHC_EWPLv5_K
  Constant5 : Constant  Value=0
  Constant6 : Constant  Value=KTHC_EWP3SpdDeice_K
  Constant7 : Constant  Value=125
  Constant8 : Constant  Value=KTHC_EWPDcCharge_K
  Multiport Switch : MultiPortSwitch  Inputs=9  DiagnosticForDefault=None
  EWPOut : Outport
  wires:
  Constant8/1 -> Multiport Switch/9
  Constant6/1 -> Multiport Switch/7
  Multiport Switch/1 -> EWPOut/1
  Constant2/1 -> Multiport Switch/4
  Constant1/1 -> Multiport Switch/3
  Constant/1 -> Multiport Switch/2
  Constant3/1 -> Multiport Switch/5
  Constant4/1 -> Multiport Switch/6
  Constant5/1 -> Multiport Switch/10
  EWPLV/1 -> Multiport Switch/1
  Constant7/1 -> Multiport Switch/8

== system thc/THC/ThermalControl/THCM_Conctrl/EWP3 ==
  EWPLV : Inport
  Constant : Constant  Value=KTHC_EWPLv1_K
  Constant1 : Constant  Value=KTHC_EWPLv2_K
  Constant2 : Constant  Value=KTHC_EWPLv3_K
  Constant3 : Constant  Value=KTHC_EWPLv4_K
  Constant4 : Constant  Value=KTHC_EWPLv5_K
  Constant5 : Constant  Value=0
  Constant6 : Constant  Value=KTHC_EWP3SpdDeice_K
  Constant7 : Constant  Value=125
  Constant8 : Constant  Value=KTHC_EWPDcCharge_K
  Multiport Switch : MultiPortSwitch  Inputs=9  DiagnosticForDefault=None
  EWPOut : Outport
  wires:
  Constant8/1 -> Multiport Switch/9
  Constant6/1 -> Multiport Switch/7
  Multiport Switch/1 -> EWPOut/1
  Constant2/1 -> Multiport Switch/4
  Constant1/1 -> Multiport Switch/3
  Constant/1 -> Multiport Switch/2
  Constant3/1 -> Multiport Switch/5
  Constant4/1 -> Multiport Switch/6
  Constant5/1 -> Multiport Switch/10
  EWPLV/1 -> Multiport Switch/1
  Constant7/1 -> Multiport Switch/8

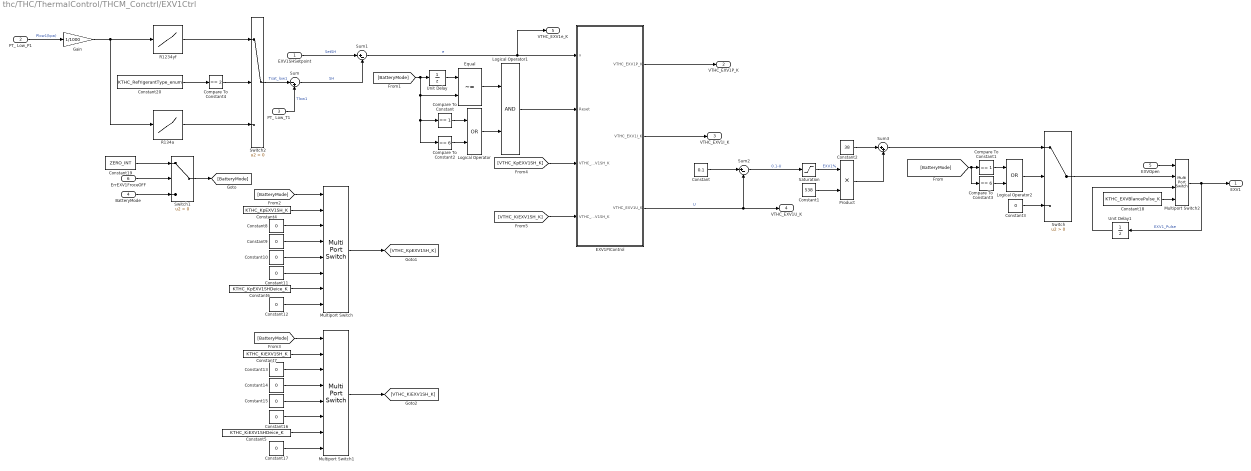
== system thc/THC/ThermalControl/THCM_Conctrl/EXV1Ctrl ==
  EXV1SHSetpoint : Inport
  PT_ Low_P1 : Inport  Port=2
  PT_ Low_T1 : Inport  Port=3
  BatteryMode : Inport  Port=4
  EXVOpen : Inport  Port=5
  ErrEXV1FroceOFF : Inport  Port=6
  Compare To Constant : simulink/Logic and Bit Operations/Compare To Constant  relop===  const=1  OutDataTypeStr=boolean
  Compare To Constant1 : simulink/Logic and Bit Operations/Compare To Constant  relop===  const=1  OutDataTypeStr=boolean
  Compare To Constant2 : simulink/Logic and Bit Operations/Compare To Constant  relop===  const=6  OutDataTypeStr=boolean
  Compare To Constant3 : simulink/Logic and Bit Operations/Compare To Constant  relop===  const=6  OutDataTypeStr=boolean
  Compare To Constant4 : simulink/Logic and Bit Operations/Compare To Constant  relop===  const=2  OutDataTypeStr=boolean
  Constant : Constant  Value=0.1
  Constant1 : Constant  Value=538
  Constant{3,8..17} (11 alike) : Constant  Value=0
  Constant18 : Constant  Value=KTHC_EXVBlancePulse_K
  Constant19 : Constant  Value=ZERO_INT
  Constant2 : Constant  Value=38
  Constant20 : Constant  Value=KTHC_RefrigerantType_enum
  Constant4 : Constant  Value=KTHC_KpEXV1SH_K
  Constant5 : Constant  Value=KTHC_KiEXV1SHDeice_K
  Constant6 : Constant  Value=KTHC_KpEXV1SHDeice_K
  Constant7 : Constant  Value=KTHC_KiEXV1SH_K
  EXV1PIControl : Subsystem
  Equal : RelationalOperator  Operator=~=  OutDataTypeStr=boolean  RndMeth=Simplest
  Gain : Gain  Gain=1/1000
  Logical Operator : Logic  Operator=OR  AllPortsSameDT=off  OutDataTypeStr=boolean
  Logical Operator1 : Logic  AllPortsSameDT=off  OutDataTypeStr=boolean
  Logical Operator2 : Logic  Operator=OR  AllPortsSameDT=off  OutDataTypeStr=boolean
  Multiport Switch : MultiPortSwitch  Inputs=7  DiagnosticForDefault=None
  Multiport Switch1 : MultiPortSwitch  Inputs=7  DiagnosticForDefault=None
  Multiport Switch2 : MultiPortSwitch  DataPortOrder=Zero-based contiguous  zeroidx=on
  Product : Product
  R1234yf : Lookup_n-D  NumberOfTableDimensions=1  BreakpointsForDimension1=[0.03742 0.06237 0.09906 0.11778 0.15092 0.1909 0.2386 0.29495 0.36092 0.43753 0.52583 0.6269 0.74189 0.87197 1.0184 1.3023]  Table=[-50 -40 -30 -26 -20 -14 -8 -2 4 10 16 22 28 34 40 50]  InternalRulePriority=Speed  RndMeth=Simplest  InputSameDT=on
  R134a : Lookup_n-D  NumberOfTableDimensions=1  BreakpointsForDimension1=[0.02945 0.05121 0.08438 0.10167 0.13273 0.17082 0.21693 0.27217 0.33766 0.41461 0.50425 0.60789 0.72688 0.86263 1.0166 1.31790]  Table=[-50 -40 -30 -26 -20 -14 -8 -2 4 10 16 22 28 34 40 50]  InternalRulePriority=Speed  RndMeth=Simplest  InputSameDT=on
  Saturation : Saturate  UpperLimit=1  LowerLimit=0
  Sum : Sum  Inputs=|-+
  Sum1 : Sum  Inputs=|+-
  Sum2 : Sum  Inputs=|+-
  Sum3 : Sum  Inputs=|++
  Switch : Switch  Criteria=u2 > Threshold
  Switch1 : Switch  Criteria=u2 > Threshold
  Switch2 : Switch  Criteria=u2 > Threshold
  Unit Delay : UnitDelay  SampleTime=-1  HasFrameUpgradeWarning=on
  Unit Delay1 : UnitDelay  SampleTime=-1  HasFrameUpgradeWarning=on
  EXV1 : Outport
  VTHC_EXV1P_K : Outport  Port=2
  VTHC_EXV1I_K : Outport  Port=3
  VTHC_EXV1U_K : Outport  Port=4
  VTHC_EXV1e_K : Outport  Port=5
  wires:
  Sum3/1 -> Switch/1
  Sum1/1 -> VTHC_EXV1e_K/1, EXV1PIControl/1(x)  "e"
  Constant1/1 -> Product/2
  [BatteryMode] -> Compare To Constant3/1, Compare To Constant1/1
  Constant3/1 -> Switch/3
  PT_ Low_P1/1 -> Gain/1  "Plow1(kpa)"
  Sum/1 -> Sum1/2  "SH"
  EXV1PIControl/3(VTHC_EXV1U_K) -> VTHC_EXV1U_K/1, Sum2/2  "U"
  Multiport Switch2/1 -> Unit Delay1/1, EXV1/1  "EXV1_Pulse"
  EXV1SHSetpoint/1 -> Sum1/1  "SetSH"
  Switch2/1 -> Sum/1  "Tsat_low1"
  Saturation/1 -> Product/1  "EXV1%"
  Product/1 -> Sum3/2
  Constant/1 -> Sum2/1
  Constant2/1 -> Sum3/1
  Sum2/1 -> Saturation/1  "0.1-U"
  PT_ Low_T1/1 -> Sum/2  "Tlow1"
  EXV1PIControl/1(VTHC_EXV1P_K) -> VTHC_EXV1P_K/1
  EXV1PIControl/2(VTHC_EXV1I_K) -> VTHC_EXV1I_K/1
  [BatteryMode] -> Unit Delay/1, Compare To Constant/1, Compare To Constant2/1, Equal/2
  Unit Delay/1 -> Equal/1
  Compare To Constant/1 -> Logical Operator/1
  Compare To Constant2/1 -> Logical Operator/2
  Equal/1 -> Logical Operator1/1
  Logical Operator/1 -> Logical Operator1/2
  Logical Operator1/1 -> EXV1PIControl/2(Reset)
  Compare To Constant1/1 -> Logical Operator2/1
  Compare To Constant3/1 -> Logical Operator2/2
  Logical Operator2/1 -> Switch/2
  [BatteryMode] -> Multiport Switch/1
  Constant4/1 -> Multiport Switch/2
  Constant6/1 -> Multiport Switch/7
  Constant5/1 -> Multiport Switch1/7
  Constant7/1 -> Multiport Switch1/2
  [BatteryMode] -> Multiport Switch1/1
  Constant8/1 -> Multiport Switch/3
  Constant9/1 -> Multiport Switch/4
  Constant10/1 -> Multiport Switch/5
  Constant11/1 -> Multiport Switch/6
  Constant12/1 -> Multiport Switch/8
  Constant13/1 -> Multiport Switch1/3
  Constant14/1 -> Multiport Switch1/4
  Constant15/1 -> Multiport Switch1/5
  Constant16/1 -> Multiport Switch1/6
  Constant17/1 -> Multiport Switch1/8
  Multiport Switch/1 -> [VTHC_KpEXV1SH_K]
  [VTHC_KpEXV1SH_K] -> EXV1PIControl/3(VTHC_KpEXV1SH_K)
  Multiport Switch1/1 -> [VTHC_KiEXV1SH_K]
  [VTHC_KiEXV1SH_K] -> EXV1PIControl/4(VTHC_KiEXV1SH_K)
  Switch/1 -> Multiport Switch2/2
  Constant18/1 -> Multiport Switch2/4
  EXVOpen/1 -> Multiport Switch2/1
  Unit Delay1/1 -> Multiport Switch2/3
  Constant19/1 -> Switch1/1
  ErrEXV1FroceOFF/1 -> Switch1/2
  Switch1/1 -> [BatteryMode]
  BatteryMode/1 -> Switch1/3
  R1234yf/1 -> Switch2/1
  Compare To Constant4/1 -> Switch2/2
  Gain/1 -> R1234yf/1, R134a/1
  R134a/1 -> Switch2/3
  Constant20/1 -> Compare To Constant4/1

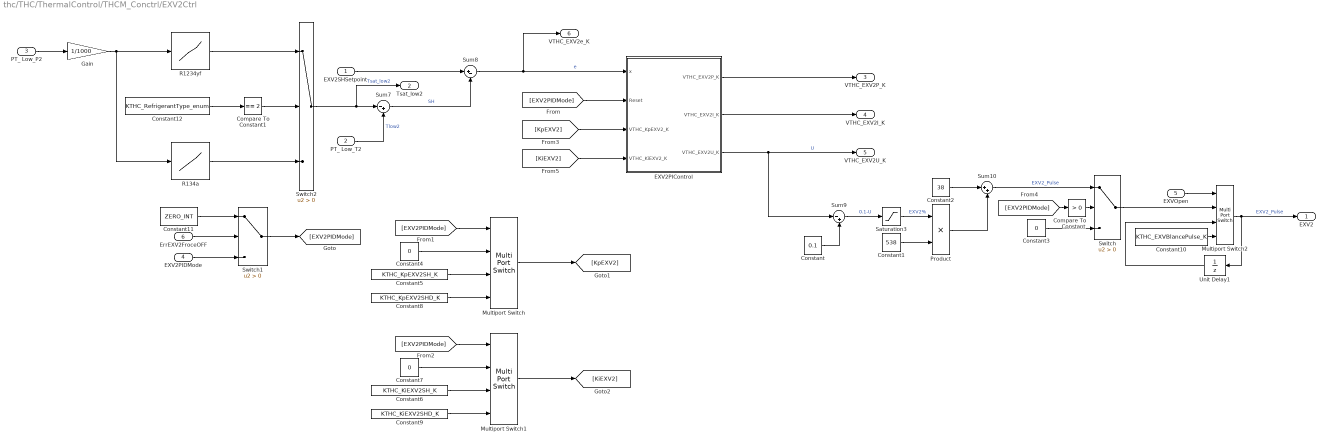
== system thc/THC/ThermalControl/THCM_Conctrl/EXV2Ctrl ==
  EXV2SHSetpoint : Inport
  PT_ Low_T2 : Inport  Port=2
  PT_ Low_P2 : Inport  Port=3
  EXV2PIDMode : Inport  Port=4
  EXVOpen : Inport  Port=5
  ErrEXV2FroceOFF : Inport  Port=6
  Compare To Constant : simulink/Logic and Bit Operations/Compare To Constant  relop=>  const=0  OutDataTypeStr=boolean
  Compare To Constant1 : simulink/Logic and Bit Operations/Compare To Constant  relop===  const=2  OutDataTypeStr=boolean
  Constant : Constant  Value=0.1
  Constant1 : Constant  Value=538
  Constant10 : Constant  Value=KTHC_EXVBlancePulse_K
  Constant11 : Constant  Value=ZERO_INT
  Constant12 : Constant  Value=KTHC_RefrigerantType_enum
  Constant2 : Constant  Value=38
  Constant3 : Constant  Value=0
  Constant4 : Constant  Value=0
  Constant5 : Constant  Value=KTHC_KpEXV2SH_K
  Constant6 : Constant  Value=KTHC_KiEXV2SH_K
  Constant7 : Constant  Value=0
  Constant8 : Constant  Value=KTHC_KpEXV2SHD_K
  Constant9 : Constant  Value=KTHC_KiEXV2SHD_K
  EXV2PIControl : Subsystem
  Gain : Gain  Gain=1/1000
  Multiport Switch : MultiPortSwitch  DataPortOrder=Zero-based contiguous  zeroidx=on
  Multiport Switch1 : MultiPortSwitch  DataPortOrder=Zero-based contiguous  zeroidx=on
  Multiport Switch2 : MultiPortSwitch  DataPortOrder=Zero-based contiguous  zeroidx=on
  Product : Product
  R1234yf : Lookup_n-D  NumberOfTableDimensions=1  BreakpointsForDimension1=[0.03742 0.06237 0.09906 0.11778 0.15092 0.1909 0.2386 0.29495 0.36092 0.43753 0.52583 0.6269 0.74189 0.87197 1.0184 1.3023]  Table=[-50 -40 -30 -26 -20 -14 -8 -2 4 10 16 22 28 34 40 50]  InternalRulePriority=Speed  RndMeth=Simplest  InputSameDT=on
  R134a : Lookup_n-D  NumberOfTableDimensions=1  BreakpointsForDimension1=[0.02945 0.05121 0.08438 0.10167 0.13273 0.17082 0.21693 0.27217 0.33766 0.41461 0.50425 0.60789 0.72688 0.86263 1.0166 1.31790]  Table=[-50 -40 -30 -26 -20 -14 -8 -2 4 10 16 22 28 34 40 50]  InternalRulePriority=Speed  RndMeth=Simplest  InputSameDT=on
  Saturation3 : Saturate  UpperLimit=1  LowerLimit=0
  Sum10 : Sum  Inputs=|++
  Sum7 : Sum  Inputs=|-+
  Sum8 : Sum  Inputs=|+-
  Sum9 : Sum  Inputs=|-+
  Switch : Switch  Criteria=u2 > Threshold
  Switch1 : Switch  Criteria=u2 > Threshold
  Switch2 : Switch  Criteria=u2 > Threshold
  Unit Delay1 : UnitDelay  SampleTime=-1  HasFrameUpgradeWarning=on
  EXV2 : Outport
  Tsat_low2 : Outport  Port=2
  VTHC_EXV2P_K : Outport  Port=3
  VTHC_EXV2I_K : Outport  Port=4
  VTHC_EXV2U_K : Outport  Port=5
  VTHC_EXV2e_K : Outport  Port=6
  wires:
  EXV2PIControl/3(VTHC_EXV2U_K) -> VTHC_EXV2U_K/1, Sum9/1  "U"
  Constant/1 -> Sum9/2
  Constant1/1 -> Product/2
  Sum9/1 -> Saturation3/1  "0.1-U"
  Gain/1 -> R1234yf/1, R134a/1
  Saturation3/1 -> Product/1  "EXV2%"
  Constant2/1 -> Sum10/1
  Sum7/1 -> Sum8/2  "SH"
  PT_ Low_T2/1 -> Sum7/2  "Tlow2"
  Sum10/1 -> Switch/1  "EXV2_Pulse"
  EXV2PIDMode/1 -> Switch1/3
  PT_ Low_P2/1 -> Gain/1
  EXV2SHSetpoint/1 -> Sum8/1
  Switch2/1 -> Tsat_low2/1, Sum7/1  "Tsat_low2"
  Sum8/1 -> VTHC_EXV2e_K/1, EXV2PIControl/1(x)  "e"
  Product/1 -> Sum10/2
  EXV2PIControl/1(VTHC_EXV2P_K) -> VTHC_EXV2P_K/1
  EXV2PIControl/2(VTHC_EXV2I_K) -> VTHC_EXV2I_K/1
  [EXV2PIDMode] -> EXV2PIControl/2(Reset)
  [EXV2PIDMode] -> Multiport Switch/1
  Constant4/1 -> Multiport Switch/2
  Constant7/1 -> Multiport Switch1/2
  [EXV2PIDMode] -> Multiport Switch1/1
  Multiport Switch/1 -> [KpEXV2]
  Constant5/1 -> Multiport Switch/3
  Constant8/1 -> Multiport Switch/4
  [KpEXV2] -> EXV2PIControl/3(VTHC_KpEXV2_K)
  Multiport Switch1/1 -> [KiEXV2]
  Constant6/1 -> Multiport Switch1/3
  Constant9/1 -> Multiport Switch1/4
  [KiEXV2] -> EXV2PIControl/4(VTHC_KiEXV2_K)
  [EXV2PIDMode] -> Compare To Constant/1
  Compare To Constant/1 -> Switch/2
  Constant3/1 -> Switch/3
  Multiport Switch2/1 -> Unit Delay1/1, EXV2/1  "EXV2_Pulse"
  Unit Delay1/1 -> Multiport Switch2/3
  EXVOpen/1 -> Multiport Switch2/1
  Constant10/1 -> Multiport Switch2/4
  Switch/1 -> Multiport Switch2/2
  ErrEXV2FroceOFF/1 -> Switch1/2
  Constant11/1 -> Switch1/1
  Switch1/1 -> [EXV2PIDMode]
  R1234yf/1 -> Switch2/1
  Constant12/1 -> Compare To Constant1/1
  Compare To Constant1/1 -> Switch2/2
  R134a/1 -> Switch2/3

== system thc/THC/ThermalControl/THCM_Conctrl/RadiatorFan ==
  FAN : Inport
  AGS_Err : Inport  Port=2
  AGS : Inport  Port=3
  Compare To Constant : simulink/Logic and Bit Operations/Compare To Constant  relop=>  const=1  OutDataTypeStr=boolean
  Constant : Constant  Value=KTHC_FANLv1_pct
  Constant1 : Constant  Value=KTHC_FANLv2_pct
  Constant2 : Constant  Value=KTHC_FANLv3_pct
  Constant3 : Constant  Value=KTHC_FANLv4_pct
  Constant4 : Constant  Value=KTHC_FANLv5_pct
  Constant5 : Constant  Value=0
  Constant6 : Constant  Value=KTHC_FANDefLv_pct
  Constant7 : Constant  Value=KTHC_ErrHandleEN_flg
  Logical Operator : Logic  Inputs=3  AllPortsSameDT=off  OutDataTypeStr=boolean
  Multiport Switch : MultiPortSwitch  Inputs=6  DiagnosticForDefault=None
  Switch : Switch  Criteria=u2 > Threshold
  CoolgFanActDuty : Outport
  wires:
  FAN/1 -> Multiport Switch/1
  Constant/1 -> Multiport Switch/2
  Constant5/1 -> Multiport Switch/7
  Constant4/1 -> Multiport Switch/6
  Constant1/1 -> Multiport Switch/3
  Constant2/1 -> Multiport Switch/4
  Constant3/1 -> Multiport Switch/5
  Logical Operator/1 -> Switch/2
  Constant6/1 -> Switch/1
  AGS/1 -> Compare To Constant/1
  AGS_Err/1 -> Logical Operator/1
  Compare To Constant/1 -> Logical Operator/2
  Switch/1 -> CoolgFanActDuty/1
  Multiport Switch/1 -> Switch/3
  Constant7/1 -> Logical Operator/3

== system thc/THC/ThermalControl/THCM_Conctrl/SensorErrorHandle1 ==
  DataIn : Inport
  SensorError : Inport  Port=2
  PresetValue : Inport  Port=3
  Constant : Constant  Value=KTHC_ErrHandleEN_flg
  Logical Operator : Logic  AllPortsSameDT=off  OutDataTypeStr=boolean
  Switch : Switch  Criteria=u2 > Threshold
  DataOut : Outport
  wires:
  PresetValue/1 -> Switch/1
  DataIn/1 -> Switch/3
  Switch/1 -> DataOut/1
  Logical Operator/1 -> Switch/2
  SensorError/1 -> Logical Operator/1
  Constant/1 -> Logical Operator/2

== system thc/THC/ThermalControl/THCM_Conctrl/SensorErrorHandle10 ==
  DataIn : Inport
  SensorError : Inport  Port=2
  PresetValue : Inport  Port=3
  Constant : Constant  Value=KTHC_ErrHandleEN_flg
  Logical Operator : Logic  AllPortsSameDT=off  OutDataTypeStr=boolean
  Switch : Switch  Criteria=u2 > Threshold
  DataOut : Outport
  wires:
  Constant/1 -> Logical Operator/2
  SensorError/1 -> Logical Operator/1
  Logical Operator/1 -> Switch/2
  Switch/1 -> DataOut/1
  DataIn/1 -> Switch/3
  PresetValue/1 -> Switch/1

== system thc/THC/ThermalControl/THCM_Conctrl/SensorErrorHandle11 ==
  DataIn : Inport
  SensorError : Inport  Port=2
  PresetValue : Inport  Port=3
  Constant : Constant  Value=KTHC_ErrHandleEN_flg
  Logical Operator : Logic  AllPortsSameDT=off  OutDataTypeStr=boolean
  Switch : Switch  Criteria=u2 > Threshold
  DataOut : Outport
  wires:
  Constant/1 -> Logical Operator/2
  SensorError/1 -> Logical Operator/1
  Logical Operator/1 -> Switch/2
  Switch/1 -> DataOut/1
  DataIn/1 -> Switch/3
  PresetValue/1 -> Switch/1

== system thc/THC/ThermalControl/THCM_Conctrl/SensorErrorHandle12 ==
  DataIn : Inport
  SensorError : Inport  Port=2
  PresetValue : Inport  Port=3
  Constant : Constant  Value=KTHC_ErrHandleEN_flg
  Logical Operator : Logic  AllPortsSameDT=off  OutDataTypeStr=boolean
  Switch : Switch  Criteria=u2 > Threshold
  DataOut : Outport
  wires:
  Constant/1 -> Logical Operator/2
  SensorError/1 -> Logical Operator/1
  Logical Operator/1 -> Switch/2
  Switch/1 -> DataOut/1
  DataIn/1 -> Switch/3
  PresetValue/1 -> Switch/1

== system thc/THC/ThermalControl/THCM_Conctrl/SensorErrorHandle2 ==
  DataIn : Inport
  SensorError : Inport  Port=2
  PresetValue : Inport  Port=3
  Constant : Constant  Value=KTHC_ErrHandleEN_flg
  Logical Operator : Logic  AllPortsSameDT=off  OutDataTypeStr=boolean
  Switch : Switch  Criteria=u2 > Threshold
  DataOut : Outport
  wires:
  Constant/1 -> Logical Operator/2
  SensorError/1 -> Logical Operator/1
  Logical Operator/1 -> Switch/2
  Switch/1 -> DataOut/1
  DataIn/1 -> Switch/3
  PresetValue/1 -> Switch/1

== system thc/THC/ThermalControl/THCM_Conctrl/SensorErrorHandle3 ==
  DataIn : Inport
  SensorError : Inport  Port=2
  PresetValue : Inport  Port=3
  Constant : Constant  Value=KTHC_ErrHandleEN_flg
  Logical Operator : Logic  AllPortsSameDT=off  OutDataTypeStr=boolean
  Switch : Switch  Criteria=u2 > Threshold
  DataOut : Outport
  wires:
  PresetValue/1 -> Switch/1
  DataIn/1 -> Switch/3
  Switch/1 -> DataOut/1
  Logical Operator/1 -> Switch/2
  SensorError/1 -> Logical Operator/1
  Constant/1 -> Logical Operator/2

== system thc/THC/ThermalControl/THCM_Conctrl/SensorErrorHandle4 ==
  DataIn : Inport
  SensorError : Inport  Port=2
  PresetValue : Inport  Port=3
  Constant : Constant  Value=KTHC_TevaErrHandleEN_flg
  Logical Operator : Logic  AllPortsSameDT=off  OutDataTypeStr=boolean
  Switch : Switch  Criteria=u2 > Threshold
  DataOut : Outport
  wires:
  PresetValue/1 -> Switch/1
  DataIn/1 -> Switch/3
  Switch/1 -> DataOut/1
  Logical Operator/1 -> Switch/2
  SensorError/1 -> Logical Operator/1
  Constant/1 -> Logical Operator/2

== system thc/THC/ThermalControl/THCM_Conctrl/SensorErrorHandle5 ==
  DataIn : Inport
  SensorError : Inport  Port=2
  PresetValue : Inport  Port=3
  Constant : Constant  Value=KTHC_TevaErrHandleEN_flg
  Logical Operator : Logic  AllPortsSameDT=off  OutDataTypeStr=boolean
  Switch : Switch  Criteria=u2 > Threshold
  DataOut : Outport
  wires:
  Constant/1 -> Logical Operator/2
  SensorError/1 -> Logical Operator/1
  Logical Operator/1 -> Switch/2
  Switch/1 -> DataOut/1
  DataIn/1 -> Switch/3
  PresetValue/1 -> Switch/1

== system thc/THC/ThermalControl/THCM_Conctrl/SensorErrorHandle6 ==
  DataIn : Inport
  SensorError : Inport  Port=2
  PresetValue : Inport  Port=3
  Constant : Constant  Value=KTHC_TevaErrHandleEN_flg
  Logical Operator : Logic  AllPortsSameDT=off  OutDataTypeStr=boolean
  Switch : Switch  Criteria=u2 > Threshold
  DataOut : Outport
  wires:
  PresetValue/1 -> Switch/1
  DataIn/1 -> Switch/3
  Switch/1 -> DataOut/1
  Logical Operator/1 -> Switch/2
  SensorError/1 -> Logical Operator/1
  Constant/1 -> Logical Operator/2

== system thc/THC/ThermalControl/THCM_Conctrl/SensorErrorHandle7 ==
  DataIn : Inport
  SensorError : Inport  Port=2
  PresetValue : Inport  Port=3
  Constant : Constant  Value=KTHC_TevaErrHandleEN_flg
  Logical Operator : Logic  AllPortsSameDT=off  OutDataTypeStr=boolean
  Switch : Switch  Criteria=u2 > Threshold
  DataOut : Outport
  wires:
  Constant/1 -> Logical Operator/2
  SensorError/1 -> Logical Operator/1
  Logical Operator/1 -> Switch/2
  Switch/1 -> DataOut/1
  DataIn/1 -> Switch/3
  PresetValue/1 -> Switch/1

== system thc/THC/ThermalControl/THCM_Conctrl/SensorErrorHandle8 ==
  DataIn : Inport
  SensorError : Inport  Port=2
  PresetValue : Inport  Port=3
  Constant : Constant  Value=KTHC_TevaErrHandleEN_flg
  Logical Operator : Logic  AllPortsSameDT=off  OutDataTypeStr=boolean
  Switch : Switch  Criteria=u2 > Threshold
  DataOut : Outport
  wires:
  PresetValue/1 -> Switch/1
  DataIn/1 -> Switch/3
  Switch/1 -> DataOut/1
  Logical Operator/1 -> Switch/2
  SensorError/1 -> Logical Operator/1
  Constant/1 -> Logical Operator/2
